simulink model "Es4_sim_nograf"  (R2017b)
settings: Solver=VariableStepAuto  StartTime=0.0  StopTime=10.0  RelTol=1e-3
values from neighbouring files (symbols this model uses):
  x0 = [10;25]    [Es4.m]
undefined symbols (not defined in the file or in its folder): e1, e2, K1, p
settings Model: Creator=claudio  LastModifiedBy=claudio

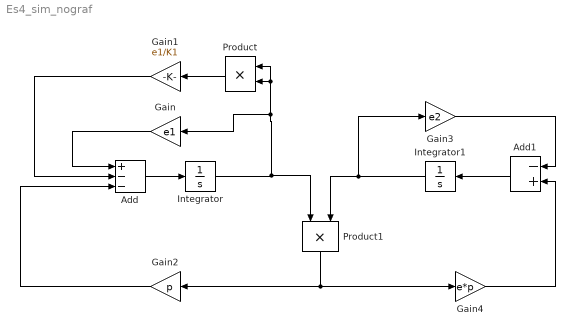
== system Es4_sim_nograf ==
  Add : Sum  Inputs=+--
  Add1 : Sum  Inputs=-+
  Gain : Gain  Gain=e1
  Gain1 : Gain  Gain=e1/K1
  Gain2 : Gain  Gain=p
  Gain3 : Gain  Gain=e2
  Gain4 : Gain  Gain=e*p
  Integrator : Integrator  InitialCondition=x0(1)
  Integrator1 : Integrator  InitialCondition=x0(2)
  Product : Product
  Product1 : Product
  wires:
  Add/1 -> Integrator/1
  Integrator/1 -> Product1/1, Gain/1, Product/1, Product/2
  Product/1 -> Gain1/1
  Gain1/1 -> Add/2
  Gain/1 -> Add/1
  Integrator1/1 -> Gain3/1, Product1/2
  Product1/1 -> Gain4/1, Gain2/1
  Gain2/1 -> Add/3
  Add1/1 -> Integrator1/1
  Gain3/1 -> Add1/1
  Gain4/1 -> Add1/2
